simulink model "fifth_equation_test_discrete"  (R2017b)
settings: Solver=VariableStepAuto  StartTime=0.0  StopTime=5  RelTol=1e-3
undefined symbols (not defined in the file): quad
libraries: NLGCToolbox x4, simulink x1
settings Model: Creator=hoang  LastModifiedBy=hoang

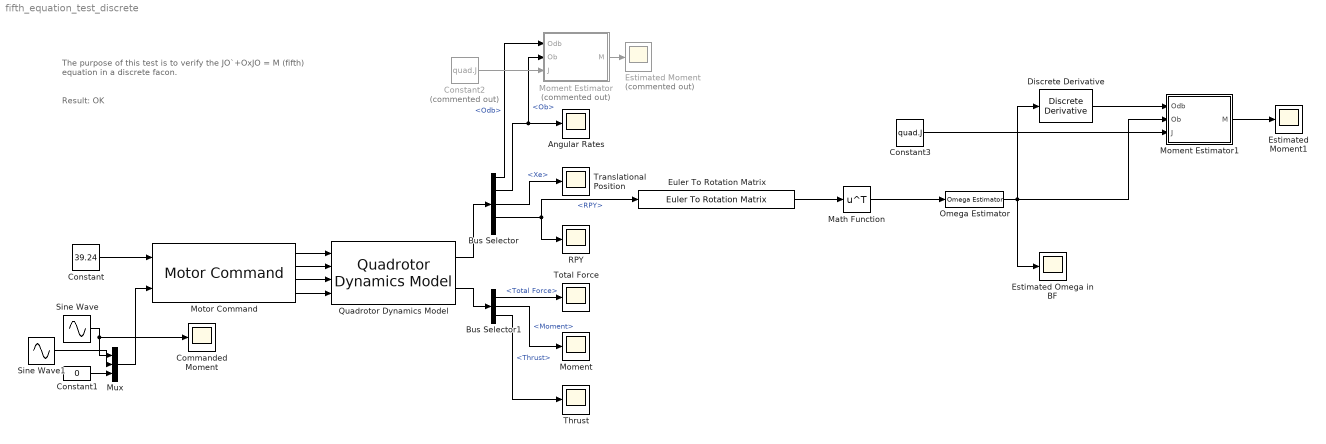
== system fifth_equation_test_discrete ==
  note: The purpose of this test is to verify the JO`+OxJO = M (fifth) equation in a discrete facon.
  note: Result: OK
  Angular Rates : Scope
  Bus Selector : BusSelector  OutputSignals=Odb,Ob,Xe,RPY,DCMbe
  Bus Selector1 : BusSelector  OutputSignals=Total Force,Moment,Thrust
  Commanded Moment : Scope
  Constant : Constant  Value=39.24
  Constant1 : Constant  Value=0
  Constant2 : Constant  Commented=on  Value=quad.J
  Constant3 : Constant  Value=quad.J
  Discrete Derivative : simulink/Discrete/Discrete Derivative  gainval=1.0  ICPrevScaledInput=0.0  OutMin=[]  OutMax=[]  OutDataType=fixdt(1, 16)  OutScaling=2^-10  DoSatur=off
  Estimated Moment : Scope  Commented=on
  Estimated Moment1 : Scope
  Estimated Omega in BF : Scope
  Euler To Rotation Matrix : NLGCToolbox/Euler To Rotation Matrix
      settings: SourceProductName=Thinh - NLGC for Quadrotor
  Math Function : Math  Operator=transpose  SaturateOnIntegerOverflow=on
  Moment : Scope
  Moment Estimator : MATLAB Function  Commented=on  TreatAsAtomicUnit=on
  Moment Estimator1 : MATLAB Function  TreatAsAtomicUnit=on
  Motor Command : NLGCToolbox/Motor Command  quadrotor=quad
      settings: SourceProductName=Thinh - NLGC for Quadrotor
  Mux : Mux  Inputs=3
  Omega Estimator : NLGCToolbox/Omega Estimator  Ts=1/120
      settings: SourceProductName=Thinh - NLGC for Quadrotor
  Quadrotor Dynamics Model : NLGCToolbox/Quadrotor Dynamics Model  xinit=[0 0 -4]  quadrotor=quad
      settings: SourceProductName=Thinh - NLGC for Quadrotor
  RPY : Scope
  Sine Wave : Sin  Amplitude=0.005  Frequency=2*pi/5  SampleTime=0
  Sine Wave1 : Sin  Amplitude=0.005  Frequency=2*pi/5  Phase=-0.12  SampleTime=0
  Thrust : Scope
  Total Force : Scope
  Translational Position : Scope
  wires:
  Motor Command/1 -> Quadrotor Dynamics Model/1
  Motor Command/2 -> Quadrotor Dynamics Model/2
  Motor Command/3 -> Quadrotor Dynamics Model/3
  Motor Command/4 -> Quadrotor Dynamics Model/4
  Constant/1 -> Motor Command/1
  Quadrotor Dynamics Model/1 -> Bus Selector/1
  Bus Selector/3 -> Translational Position/1  "<Xe>"
  Bus Selector/4 -> RPY/1, Euler To Rotation Matrix/1  "<RPY>"
  Quadrotor Dynamics Model/2 -> Bus Selector1/1
  Bus Selector1/1 -> Total Force/1  "<Total Force>"
  Bus Selector1/2 -> Moment/1  "<Moment>"
  Mux/1 -> Motor Command/2
  Sine Wave/1 -> Commanded Moment/1, Mux/1
  Bus Selector1/3 -> Thrust/1  "<Thrust>"
  Constant1/1 -> Mux/3
  Bus Selector/2 -> Moment Estimator/2(Ob), Angular Rates/1  "<Ob>"
  Bus Selector/1 -> Moment Estimator/1(Odb)  "<Odb>"
  Moment Estimator/1(M) -> Estimated Moment/1
  Constant2/1 -> Moment Estimator/3(J)
  Omega Estimator/1 -> Moment Estimator1/2(Ob), Estimated Omega in BF/1, Discrete Derivative/1
  Euler To Rotation Matrix/1 -> Math Function/1
  Math Function/1 -> Omega Estimator/1
  Sine Wave1/1 -> Mux/2
  Discrete Derivative/1 -> Moment Estimator1/1(Odb)
  Constant3/1 -> Moment Estimator1/3(J)
  Moment Estimator1/1(M) -> Estimated Moment1/1

== matlab function fifth_equation_test_discrete/Moment Estimator1 ==
  data: M output size=[3 1]; Odb input size=[3 1]; Ob input size=[3 1]; J input size=[3 3]
function M = fcn(Odb,Ob,J)
M = J*Odb + hat(Ob)*(J*Ob);

== matlab function fifth_equation_test_discrete/Moment Estimator ==
  data: M output size=[3 1]; Odb input size=[3 1]; Ob input size=[3 1]; J input size=[3 3]
function M = fcn(Odb,Ob,J)
M = J*Odb + hat(Ob)*(J*Ob);
